simulink model "SimulinkMorphEUS"  (R2025a)
settings: Solver=VariableStepAuto  StartTime=0.0  StopTime=Tfinal  RelTol=1e-3
values from neighbouring files (symbols this model uses):
  Ixx = 0.246    [SetDroneControl(5).m]    (also in SetDroneControl.m)
  Iyy = 0.336    [SetDroneControl(5).m]    (also in SetDroneControl.m)
  Izz = 0.234    [SetDroneControl(5).m]    (also in SetDroneControl.m)
  lx = 0.2125    [SetDroneControl(5).m]    (also in SetDroneControl.m)
  ly = 0.2125    [SetDroneControl(5).m]    (also in SetDroneControl.m)
  Mass = 3    [SetDroneControl(5).m]    (also in SetDroneControl.m = 5)
libraries: slpidlib x12, matrix_library x8, robotcorelib x4, aerolibobsolete x1, uavutilslib x1
(part 2 of 2)

== matlab function SimulinkMorphEUS/Subsystem1/MATLAB Function3 ==
  data: fd input; Omega output; tau input; alpha output; beta output
function [Omega, alpha, beta] = controlAllocation(fd, tau)
% Compute thrust allocation for vectored-thrust quadrotor
% Inputs:
%   fd   - desired total thrust (scalar)
%   tau  - desired torques [tau_x; tau_y; tau_z]
%   lx, ly - half-length, half-breadth
%   ct   - coefficient relating Omega^2 to thrust magnitude
kB = [0;0;1];
lx = 0.2125;
ly = 0.2125;
ct = 0.013;
% Outputs:
%   Omega - 4x1 rotor speeds
%   alpha - 4x1 tilt angle alpha_i
%   beta  - 4x1 tilt angle beta_i
%   t     - 3x4 thrust vectors (each column is t_i)

tau_x = tau(1); tau_y = tau(2); tau_z = tau(3);
r = sqrt(lx^2 + ly^2);

% Unit yaw vectors (eq. 12)
tpsi1 = [-ly/r;  lx/r; 0];
tpsi2 = [ ly/r;  lx/r; 0];
tpsi3 = [ ly/r; -lx/r; 0];
tpsi4 = [-ly/r; -lx/r; 0];

% Thrust vector for each rotor (eq. 11)
t = zeros(3,4);
t(:,1) = fd/4 + ( tau_x/(4*ly) )*kB + (-tau_y/(4*lx))*kB + (tau_z/(4*r))*tpsi1;
t(:,2) = fd/4 + (-tau_x/(4*ly))*kB + (-tau_y/(4*lx))*kB + (tau_z/(4*r))*tpsi2;
t(:,3) = fd/4 + (-tau_x/(4*ly))*kB + ( tau_y/(4*lx))*kB + (tau_z/(4*r))*tpsi3;
t(:,4) = fd/4 + ( tau_x/(4*ly) )*kB + ( tau_y/(4*lx))*kB + (tau_z/(4*r))*tpsi4;

% Initialize outputs
Omega = zeros(4,1);
alpha = zeros(4,1);
beta  = zeros(4,1);

% For each rotor compute Omega, beta, alpha (eq. 14–15)
for i = 1:4
    ti = t(:,i);
    ti_norm = norm(ti);
    if ti_norm < 1e-6
        Omega(i) = 0; alpha(i) = 0; beta(i) = 0;
        continue;
    end
    
    % normalized thrust vector
    that = ti / ti_norm;
    
    % Rotor speed
    Omega(i) = sqrt(ti_norm/ct);
    
    % beta (tilt around y-axis)
    beta(i) = -asin(that(2));
    
    % alpha (tilt around x-axis), depends on quadrant (eq. 15)
    if ti(3) < 0 && ti(1) >= 0
        alpha(i) = pi - asin(that(1)/cos(beta(i)));
    elseif ti(3) < 0 && ti(1) < 0
        alpha(i) = -pi - asin(that(1)/cos(beta(i)));
    else
        alpha(i) = asin(that(1)/cos(beta(i)));
    end
end
end

== matlab function SimulinkMorphEUS/MATLAB Function ==
  data: clock input; mode output
function mode = fcn(clock)
if clock < 1
    mode = 0;
else
    mode = 1  ;  
end
